simulink model "density"  (R2021a)
settings: Solver=VariableStepAuto  StartTime=0.0  StopTime=10.0  RelTol=1e-3
values from neighbouring files (symbols this model uses):
  g_0 = 9.798    [main_simulation.m]
  H_0 = 7249000    [main_simulation.m]
  h_0 = 0    [main_simulation.m]
  m_0 = 74 * lb2kg    (= 33.56583538)    [main_simulation.m]
  R_E = 6378136    [main_simulation.m]
  rho_0 = 1.225    [main_simulation.m]
  t_BO = 6.3    [main_simulation.m]
undefined symbols (not defined in the file or in its folder): Theta_0
settings Model: Creator=SeverinBeger  LastModifiedBy=SeverinBeger

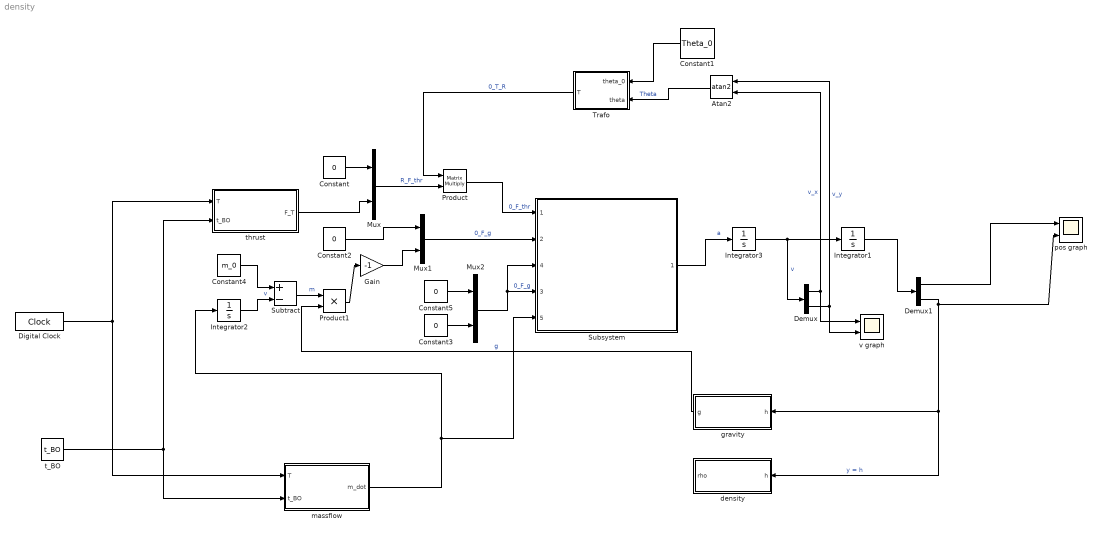
== system density ==
  Atan2 : Trigonometry  Operator=atan2
  Constant{,2..3,5} (4 alike) : Constant  Value=0
  Constant1 : Constant  Value=Theta_0
  Constant4 : Constant  Value=m_0
  Demux : Demux  Outputs=2
  Demux1 : Demux  Outputs=2
  Digital Clock : DigitalClock
  Gain : Gain  Gain=-1
  Integrator1 : Integrator
  Integrator2 : Integrator
  Integrator3 : Integrator
  Mux : Mux  Inputs=2
  Mux1 : Mux  Inputs=2
  Mux2 : Mux  Inputs=2
  Product : Product  Multiplication=Matrix(*)
  Product1 : Product
  Subsystem : Subsystem  ReferencedSubsystem=acceleration
      settings: PortSchema="{\"entries\":[{\"content\":{\"sides\":[{\"content\":{\"connectorIds\":[\"In1\",\"In2\",\"In4\",\"In3\",\"In5\"]},\"type\":\"ConnectorPlacement.EquallySpacedRectSide\",\"uuid\":\"9ef3e48b-891b-4d0d-a708-ee121c0097dd\"},{\"content\":{\"connectorIds\":[\"Out1\"],\"side\":\"RIGHT\"},\"type\":\"ConnectorPlacement.EquallySpacedRectSide\",\"uuid\":\"fe012b3b-856e-4c20-af45-176b50db60e5\"},{\"content\":{\"connectorIds\":[],\"side\":\"TOP\"},\"type\":\"ConnectorPlacement.EquallySpacedRectSide\",\"uuid\":\"c344a42b-cb7d-481a-b552-86bd89250f10\"}]},\"type\":\"ConnectorPlacement.EquallySpacedConnector\",\"uuid\":\"b7d8efea-7233-4c8a-80e4-a1935eebb6ed\"}],\"packageUris\":[\"http://schema.mathworks.com/mf0/Connector/R2020b\"],\"version\":\"1.0\"}"
  Subtract : Sum  Inputs=+-
  Trafo : MATLAB Function  TreatAsAtomicUnit=on
  density : Subsystem
  gravity : Subsystem
  massflow : MATLAB Function  TreatAsAtomicUnit=on
  pos graph : Scope  NumInputPorts=2
  t_BO : Constant  Value=t_BO
  thrust : MATLAB Function  TreatAsAtomicUnit=on
  v graph : Scope  NumInputPorts=2
  wires:
  Subsystem/1 -> Integrator3/1  "a"
  Integrator3/1 -> Integrator1/1, Demux/1  "v"
  Integrator1/1 -> Demux1/1
  Demux1/2 -> gravity/1(h), density/1(h), pos graph/2  "y = h"
  massflow/1(m_dot) -> Integrator2/1, Subsystem/5
  t_BO/1 -> massflow/2(t_BO), thrust/2(t_BO)
  Digital Clock/1 -> massflow/1(T), thrust/1(T)
  Demux/2 -> Atan2/1, v graph/2  "v_y"
  Demux/1 -> Atan2/2, v graph/1  "v_x"
  Atan2/1 -> Trafo/2(theta)  "Theta"
  thrust/1(F_T) -> Mux/2
  Constant/1 -> Mux/1
  Product/1 -> Subsystem/1  "0_F_thr"
  Mux/1 -> Product/2  "R_F_thr"
  Trafo/1(T) -> Product/1  "0_T_R"
  Constant1/1 -> Trafo/1(theta_0)
  Constant2/1 -> Mux1/1
  Mux1/1 -> Subsystem/2  "0_F_g"
  Integrator2/1 -> Subtract/2  "v"
  Constant4/1 -> Subtract/1
  Product1/1 -> Gain/1
  Gain/1 -> Mux1/2
  Subtract/1 -> Product1/1  "m"
  gravity/1(g) -> Product1/2  "g"
  Constant5/1 -> Mux2/1
  Constant3/1 -> Mux2/2
  Mux2/1 -> Subsystem/3, Subsystem/4  "0_F_g"
  Demux1/1 -> pos graph/1

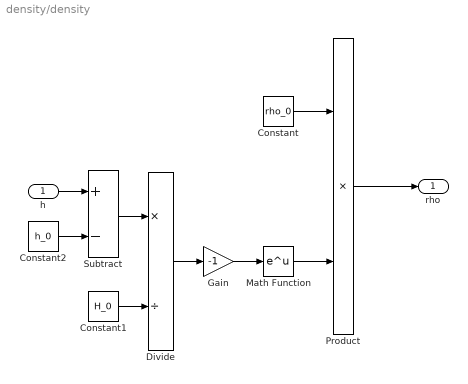
== system density/density ==
  h : Inport
  Constant : Constant  Value=rho_0  VectorParams1D=off
  Constant1 : Constant  Value=H_0  VectorParams1D=off
  Constant2 : Constant  Value=h_0  VectorParams1D=off
  Divide : Product  Inputs=*/
  Gain : Gain  Gain=-1
  Math Function : Math  SaturateOnIntegerOverflow=on
  Product : Product
  Subtract : Sum  Inputs=+-
  rho : Outport
  wires:
  h/1 -> Subtract/1
  Constant2/1 -> Subtract/2
  Subtract/1 -> Divide/1
  Constant1/1 -> Divide/2
  Divide/1 -> Gain/1
  Gain/1 -> Math Function/1
  Math Function/1 -> Product/2
  Constant/1 -> Product/1
  Product/1 -> rho/1

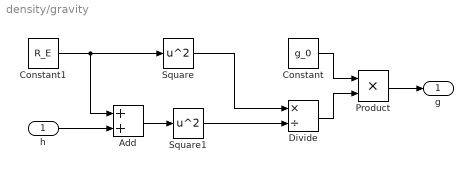
== system density/gravity ==
  h : Inport
  Add : Sum
  Constant : Constant  Value=g_0
  Constant1 : Constant  Value=R_E
  Divide : Product  Inputs=*/
  Product : Product
  Square : Math  Operator=square  SaturateOnIntegerOverflow=on
  Square1 : Math  Operator=square  SaturateOnIntegerOverflow=on
  g : Outport
  wires:
  h/1 -> Add/2
  Constant1/1 -> Square/1, Add/1
  Add/1 -> Square1/1
  Square/1 -> Divide/1
  Square1/1 -> Divide/2
  Divide/1 -> Product/2
  Constant/1 -> Product/1
  Product/1 -> g/1

== matlab function density/massflow ==
  data: T input; m_dot output; t_BO input
function m_dot = massflow(T,t_BO)
% this is an interpolation of the massflow for a certain rocket motor:
% O3400
%Inputs: Time T to evaluate, time of burnout of motort
%Output: massflow at time T in kg:  m_dot(T)
m_dot = 0;
if(T <= t_BO)
    %data:
    t = [0, 0.04, 0.052, 0.101, 0.19, 0.38, 0.965, 2.176, 2.887,3.658, 4.17, 4.493, ...
        4.881, 5.483, 6.137, 6.322];
    m = 1e-3.*[11272, 11229.6, 11202.6, 11085.2, 10872.1, 10423.7, 9039.12, 6073.35, 4303.95,...
        2482.87,1511.85,1043.46, 609.199, 207.979, 12.3006, 0];

    m_dot_arr = [0];

    for i=2:length(t)
        m_dot_arr = [m_dot_arr, (m(i)-m(i-1))/(t(i)-t(i-1))];
    end

    % interpolate:
    t_delta = T-t;
    [min_t,idx] = min(abs(t_delta));
    
    if t_delta(idx) < 0
        p1 = idx-1;
        p2 = idx;
    elseif min_t > 0
        p1 = idx;
        p2 = idx + 1;
    else
        m_dot = m_dot_arr(idx);
        return;
    end
    
    m_dot = m_dot_arr(p1) + (m_dot_arr(p2)-m_dot_arr(p1))*(T-t(p1))/(t(p2)-t(p1));
end
end

== matlab function density/Trafo ==
  data: theta_0 input; theta input; T output
function T = Trafo(theta_0,theta)
 %Transformation from the rocket coordinate system to the world system
 %(x,y)
 if(isnan(theta))
     theta = theta_0;
 end
 T = [cos(theta), -sin(theta);
     sin(theta),cos(theta)];
endfunction y = fcn(u)

y = u;

== matlab function density/thrust ==
  data: T input; F_T output; t_BO input
function F_T = thrust(T,t_BO)
% this is an interpolation of the thrust for a certain rocket motor:
% O3400
%Inputs: Time T to evaluate, time of burnout of motort
%Output: thrust at time T in N:  F_T(T)
F_T = 0;
    if(T <= t_BO)
        %data:
        t = [0, 0.04, 0.052, 0.101, 0.19, 0.38, 0.965, 2.176, 2.887,3.658, 4.17, 4.493, ...
            4.881, 5.483, 6.137, 6.322];
        f = [0, 3959.81, 4432.62, 4515.37, 4420.8, 4391.25, 4444.44, 4698.58, 4592.2, 4225.77,...
            2854.61, 2559.1, 1619.38, 868.794, 248.227, 0];


        % interpolate:
        t_delta = T-t;
        [min_t,idx] = min(abs(t_delta));

        if t_delta(idx) < 0
            p1 = idx-1;
            p2 = idx;
        elseif min_t > 0
            p1 = idx;
            p2 = idx + 1;
        else
            F_T = f(idx);
            return;
        end

        F_T = f(p1) + (f(p2)-f(p1))*(T-t(p1))/(t(p2)-t(p1));
    end
end
